simulink model "sauna_sim"  (R2023a)
settings: Solver=VariableStepAuto  StartTime=0.0  StopTime=3600*2  RelTol=1e-3  AbsTol=1e-3
undefined symbols (not defined in the file or in its folder): cost_electricity, cost_gas, gebouw2_temp, gebouw_temp, mean_mean, opgiet_deur_d, opgiet_deur_opp, opgiet_muur_1_hout_d, opgiet_muur_1_isol_d, opgiet_muur_1_opp, opgiet_muur_2_opp, opgiet_muur_3_opp, opgiet_muur_4_opp, opgiet_plafond_opp, opgiet_volume, R_hout, R_hout_plafond, R_isol, R_muur_2_gips, R_muur_3_gips, R_muur_3_raam, R_muur_4_buiten, R_muur_4_gips, R_muur_4_raam, R_opgiet_hout, R_opgiet_isol, R_sauna2_deur, R_se, R_si, rho_lucht, sauna1_deur_d, sauna1_deur_opp, sauna1_muur_1_hout_d, sauna1_muur_1_isol_d, sauna1_muur_1_opp, sauna1_muur_2_gips_d, sauna1_muur_2_opp, sauna1_muur_3_gips_d, sauna1_muur_3_opp, sauna1_muur_4_gips_d, sauna1_muur_4_opp, sauna1_plafond_hout_d, sauna1_plafond_isol_d, sauna1_plafond_opp, sauna1_R_muur_2_gips, sauna1_R_muur_3_gips, sauna1_R_muur_4_gips, sauna1_vol, sauna2_deur_opp, sauna2_muur_1_hout_d, sauna2_muur_1_isol_d, sauna2_muur_1_opp, sauna2_muur_2_gips_d, sauna2_muur_2_opp, sauna2_muur_3_gips_d, sauna2_muur_3_opp, sauna2_muur_3_raam_d, sauna2_muur_3_raam_opp, sauna2_muur_4_gips_d, sauna2_muur_4_opp ... (+6)
libraries: fl_lib x491, nesl_utility x30
(part 2 of 6)

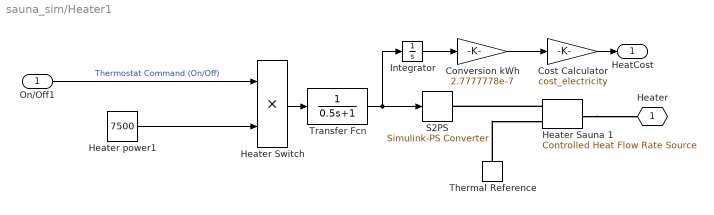
== system sauna_sim/Heater1 ==
  On/Off1 : Inport
  Conversion kWh : Gain  Gain=2.7777778e-7  SaturateOnIntegerOverflow=on  OutDataTypeStr=Inherit: Same as input  ParamDataTypeStr=Inherit: Same as input
  Cost Calculator : Gain  Gain=cost_electricity  SaturateOnIntegerOverflow=on  OutDataTypeStr=Inherit: Same as input  ParamDataTypeStr=Inherit: Same as input
  Heater Sauna 1 : fl_lib/Thermal/Thermal Sources/Controlled Heat Flow Rate Source
  Heater Switch : Product  RndMeth=Zero
  Heater power1 : Constant  Value=7500
  Integrator : Integrator
  S2PS : nesl_utility/Simulink-PS Converter  PhysicalDomain=network_engine_domain  SubClassName=ps_input  LeftPortType=input  RightPortType=output  PseudoPeriodic=off  Frequencies=[]  NoiseDistribution=none  NoiseParameters=[]  Unit=1  AffineConversion=off  FilteringAndDerivatives=zero  SimscapeFilterOrder=1  InputFilterTimeConstant=.001  UdotUserProvided=0
  Thermal Reference : fl_lib/Thermal/Thermal Elements/Thermal Reference
  Transfer Fcn : TransferFcn  Denominator=[0.5 1]
  Heater : PMIOPort  Tag=PMCPort  Side=Right
  HeatCost : Outport  VectorParamsAs1DForOutWhenUnconnected=off
  wires:
  Cost Calculator/1 -> HeatCost/1
  Heater Switch/1 -> Transfer Fcn/1
  Integrator/1 -> Conversion kWh/1
  Conversion kWh/1 -> Cost Calculator/1
  Transfer Fcn/1 -> S2PS/1, Integrator/1
  Heater power1/1 -> Heater Switch/2
  On/Off1/1 -> Heater Switch/1  "Thermostat Command (On/Off)"
  connections:
  Heater Sauna 1/RConn1 -- S2PS/RConn1
  Thermal Reference/LConn1 -- Heater Sauna 1/RConn2
  Heater Sauna 1/LConn1 -- Heater/RConn1

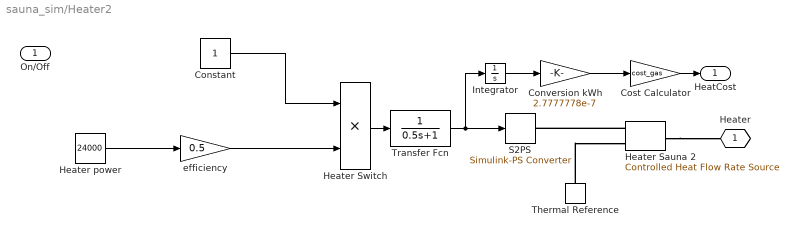
== system sauna_sim/Heater2 ==
  On/Off : Inport
  Constant : Constant
  Conversion kWh : Gain  Gain=2.7777778e-7  SaturateOnIntegerOverflow=on  OutDataTypeStr=Inherit: Same as input  ParamDataTypeStr=Inherit: Same as input
  Cost Calculator : Gain  Gain=cost_gas  SaturateOnIntegerOverflow=on  OutDataTypeStr=Inherit: Same as input  ParamDataTypeStr=Inherit: Same as input
  Heater Sauna 2 : fl_lib/Thermal/Thermal Sources/Controlled Heat Flow Rate Source
  Heater Switch : Product  RndMeth=Zero
  Heater power : Constant  Value=24000
  Integrator : Integrator
  S2PS : nesl_utility/Simulink-PS Converter  PhysicalDomain=network_engine_domain  SubClassName=ps_input  LeftPortType=input  RightPortType=output  PseudoPeriodic=off  Frequencies=[]  NoiseDistribution=none  NoiseParameters=[]  Unit=1  AffineConversion=off  FilteringAndDerivatives=zero  SimscapeFilterOrder=1  InputFilterTimeConstant=.001  UdotUserProvided=0
  Thermal Reference : fl_lib/Thermal/Thermal Elements/Thermal Reference
  Transfer Fcn : TransferFcn  Denominator=[0.5 1]
  efficiency : Gain  Gain=0.5  SaturateOnIntegerOverflow=on  OutDataTypeStr=Inherit: Same as input  ParamDataTypeStr=Inherit: Same as input
  Heater : PMIOPort  Tag=PMCPort  Side=Right
  HeatCost : Outport  VectorParamsAs1DForOutWhenUnconnected=off
  wires:
  Cost Calculator/1 -> HeatCost/1
  Heater Switch/1 -> Transfer Fcn/1
  Heater power/1 -> efficiency/1
  Integrator/1 -> Conversion kWh/1
  Conversion kWh/1 -> Cost Calculator/1
  Transfer Fcn/1 -> S2PS/1, Integrator/1
  Constant/1 -> Heater Switch/1
  efficiency/1 -> Heater Switch/2
  connections:
  Heater Sauna 2/RConn1 -- S2PS/RConn1
  Thermal Reference/LConn1 -- Heater Sauna 2/RConn2
  Heater Sauna 2/LConn1 -- Heater/RConn1
